simulink model "noise"  (R2022b)
settings: Solver=VariableStepAuto  StartTime=0.0  StopTime=1000  RelTol=1e-3
values from neighbouring files (symbols this model uses):
  dataToSimulink = [time, myData]    [jelob.m]
libraries: dsparch4 x3, dspstat3 x1
settings Model: Creator=admin  LastModifiedBy=anver
settings DebuggingCC: UnconnectedInputMsg=warning  UnconnectedOutputMsg=warning  UnconnectedLineMsg=warning
settings ModelReferenceCC: EnableRefExpFcnMdlSchedulingChecks=on
settings RTWCC: DLArmComputeVersion=19.05

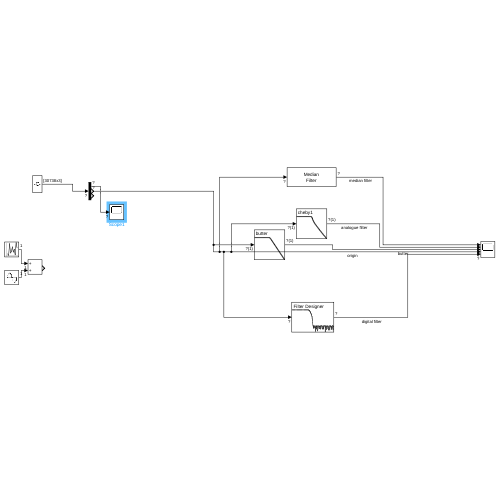
[thumbnail: Simulink's stored preview of the top-level diagram]
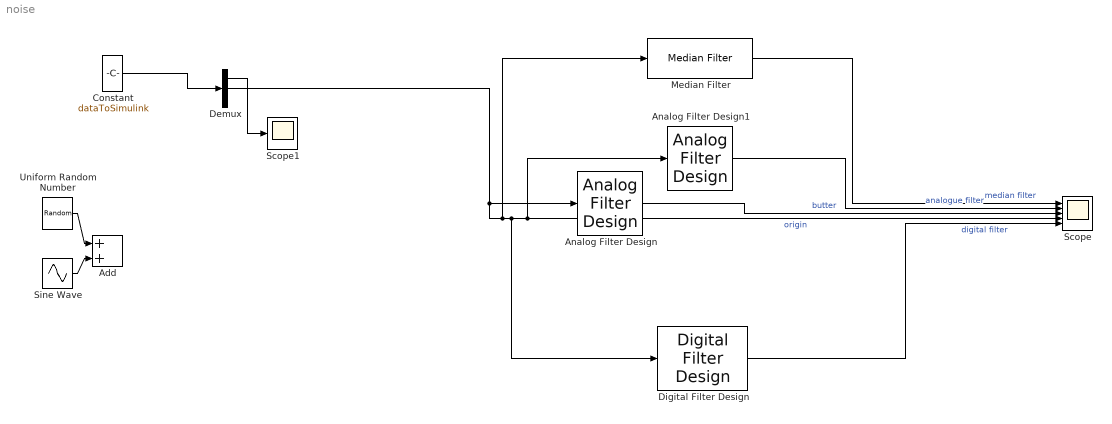
== system noise ==
  Add : Sum
  Analog Filter Design : dsparch4/Analog Filter Design  method=Butterworth  filttype=Lowpass  N=10  Wlo=30  Whi=80  Rp=2  Rs=40
  Analog Filter Design1 : dsparch4/Analog Filter Design  method=Chebyshev I  filttype=Lowpass  N=8  Wlo=0.0006  Whi=80  Rp=2  Rs=40
  Constant : Constant  Value=dataToSimulink
  Demux : Demux  Outputs=3
  Digital Filter Design : dsparch4/Digital Filter Design  mwdsp_browser_bugfix_var=off
  Median Filter : dspstat3/Median Filter  WindowLength=10000  SimulateUsing=Code generation
  Scope : Scope  NumInputPorts=5
  Scope1 : Scope
  Sine Wave : Sin  SampleTime=0.1
  Uniform Random Number : UniformRandomNumber  SampleTime=0.1
  wires:
  Analog Filter Design1/1 -> Scope/2  "analogue filter"
  Median Filter/1 -> Scope/1  "median filter"
  Digital Filter Design/1 -> Scope/5  "digital filter"
  Demux/2 -> Median Filter/1, Digital Filter Design/1, Analog Filter Design1/1, Scope/4, Analog Filter Design/1  "origin"
  Sine Wave/1 -> Add/2
  Uniform Random Number/1 -> Add/1
  Analog Filter Design/1 -> Scope/3  "butter"
  Constant/1 -> Demux/1
  Demux/1 -> Scope1/1
